simulink model "A"  (Simulink 8.8)
settings: Solver=ode4  StartTime=0.0  StopTime=inf  FixedStep=0.001  RelTol=1e-3  EnableMultiTasking=on
undefined symbols (not defined in the file): mdaadlink6208
settings Model: Creator=Tao  LastModifiedBy=youcaihua  SimulationMode=external
settings SolverCC: EnableConcurrentExecution=on
settings DataIOCC: SaveFormat=StructureWithTime
settings OptimizationCC: BlockReduction=off  OptimizeBlockIOStorage=off  BufferReuse=off  GlobalBufferReuse=off  ExpressionFolding=off  ExpressionDepthLimit=2147483647  LocalBlockOutputs=off  LifeSpan=auto
settings DebuggingCC: SolverPrmCheckMsg=warning
settings HardwareCC: ProdIntDivRoundTo=Zero  ProdEndianess=LittleEndian  ProdLongLongMode=on  ProdHWDeviceType=Generic->32-bit x86 compatible
settings RTWCC: SystemTargetFile=slrt.tlc  TemplateMakefile=slrt_default_tmf  Description=Simulink Real-Time  RTWCompilerOptimization=on

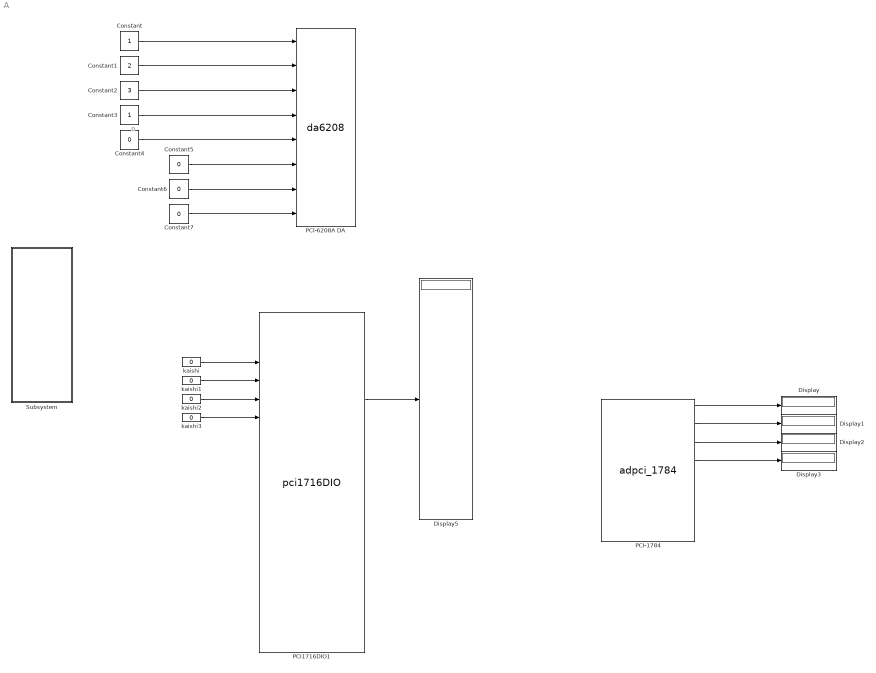
== system A ==
  note: 0
  Constant : Constant
  Constant1 : Constant  Value=2
  Constant2 : Constant  Value=3
  Constant3 : Constant
  Constant{4..7} (4 alike) : Constant  Value=0
  Display{,1..3,5} (5 alike) : Display
  PCI-1784 : S-Function  FunctionName=adpci_1784  Parameters=channel, sampletime, slot  SFunctionDeploymentMode=off  EnableBusSupport=off  mask(PCI-1784){channel=[1 2 3 4 5 6 7 8], sampletime=-1, slot=-1}
      mask prompts: channel "Channel vector:"; sampletime "Sample time:"; slot "PCI slot:"
      mask help:
      | YANHUA
      | PCI-1784
      | Motor Counter
      | UESTC
      mask init:
      | [maskdisplay] = mCntPCI_1784(channel, slot);
      | set_param( gcb, 'MaskDisplay', maskdisplay );
      settings: CopyFcn=|
      | if ~strcmp(get_param(gcb,'Linkstatus'),'none') && ...
      | ~strcmp(get_param(gcb,'Linkstatus'),'implicit')
      |   set_param(gcb,'LinkStatus','none');
      | end
      mask Display: disp('PCI-1784\nUESTC\nMotor Counter');port_label('output',1,'Cnt1');port_label('output',2,'Cnt2');port_label('output',3,'Cnt3');port_label('output',4,'Cnt4');port_label('output',5,'Index1');port_label('output',6,'Index2');port_label('output',7,'Index3');port_label('output',8,'Index4');
  "PCI-6208A DA " : S-Function  InitFcn=mdaadlink6208( 1 );  FunctionName=da6208  Parameters=channel, range, sampletime, pcislot, reset, initval  SFunctionDeploymentMode=off  EnableBusSupport=off  mask(da6208){channel=[1:8], range=4 to 20 ma, reset=[0], initval=[0], sampletime=-1, pcislot=-1}
      mask prompts: channel "Channel vector:"; reset "Reset vector:"; initval "Initial value vector:"; sampletime "Sample time:"; pcislot "PCI slot (-1: autosearch):"
      mask help:
      | PCI-6208A
      | Adlink
      | Analog Output
      mask init:
      | [maskdisplay, reset, initval]= mdaadlink6208(2, channel, reset, initval, pcislot);
      | set_param(gcb,'MaskDisplay',maskdisplay);
      mask Help: helpview(fullfile(docroot, 'mapfiles', 'xpc.map'), 'Adlink_6208A_DA')
      mask TypeOptions range: 0 to 20 ma | 5 to 25 ma | 4 to 20 ma
      mask Display: disp('PCI-6208A\nAdlink\nAnalog Output');port_label('input',1,'1');port_label('input',2,'2');port_label('input',3,'3');port_label('input',4,'4');port_label('input',5,'5');port_label('input',6,'6');port_label('input',7,'7');port_label('input',8,'8');
  PCI1716DIO1 : S-Function  FunctionName=pci1716DIO  Parameters=[SampleTime SampleOffset], SLOT  SFunctionDeploymentMode=off  EnableBusSupport=off  mask{Sample=-1, SLOT=[2 12]}
      mask prompts: Sample "Sample Time:"
      mask help:
      | PCI1716DIO
      | A/D Card
      | Harbin
      | 2014.06.06
      mask init:
      | SampleTime = -1; SampleOffset=0;
      mask Display:
      | disp('PCI1716   A/D&D/A&DIO  ');
      | port_label('input',1 , 'IN1');
      | port_label('input',2 , 'IN2');
      | port_label('input',3 , 'D1');
      | port_label('input',4 , 'D2');
      | port_label('input',5 , 'D3');
      | port_label('input',6 , 'D4');
      | port_label('input',7 , 'D5');
      | port_label('input',8 , 'D6');
      | port_label('input',9 , 'D7');
      | port_label('input',10 , 'D8');
      | port_label('input',11 , 'D9');
      | port_label('input',12 , 'D10');
      | port_label('input',13 , 'D11');
      | port_label('input',14 , 'D12');
      | port_label('input',15 , 'D13');
      | port_label('input',16 , 'D14');
      | port_label('input',17 , 'D15');
      | port_label('input',18, 'D16');
      | port_label('output',1 , 'AD(16)');
      | port_label('output',2 , 'D_OUT(16)');
  Subsystem : Subsystem
  kaishi{,1..3} (4 alike) : Constant  Value=0
      settings: OpenFcn=|
      | if get_param(gcb,'value')=='1',
      | set_param(gcb,'value','0');
      | else
      | set_param(gcb,'value','1');end
  wires:
  PCI-1784/1 -> Display/1
  PCI-1784/2 -> Display1/1
  PCI-1784/3 -> Display2/1
  PCI-1784/4 -> Display3/1
  kaishi/1 -> PCI1716DIO1/3
  kaishi1/1 -> PCI1716DIO1/4
  kaishi2/1 -> PCI1716DIO1/5
  kaishi3/1 -> PCI1716DIO1/6
  PCI1716DIO1/1 -> Display5/1
  Constant/1 -> "PCI-6208A DA "/1
  Constant4/1 -> "PCI-6208A DA "/5
  Constant5/1 -> "PCI-6208A DA "/6
  Constant6/1 -> "PCI-6208A DA "/7
  Constant7/1 -> "PCI-6208A DA "/8
  Constant1/1 -> "PCI-6208A DA "/2
  Constant2/1 -> "PCI-6208A DA "/3
  Constant3/1 -> "PCI-6208A DA "/4

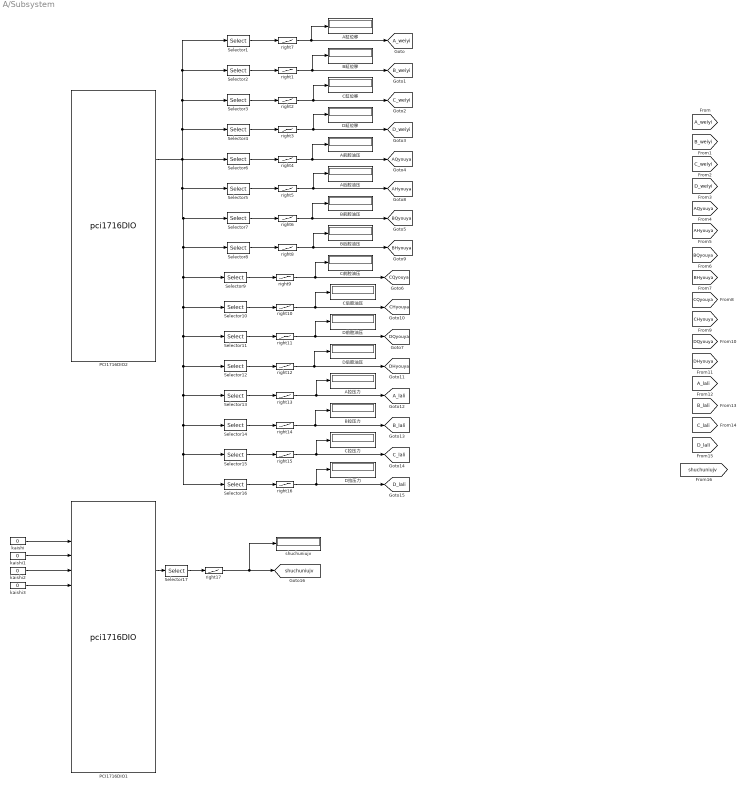
== system A/Subsystem ==
  A前腔油压 : Display
  A后腔油压 : Display
  A拉压力 : Display
  A缸位移 : Display
  B前腔油压 : Display
  B后腔油压 : Display
  B拉压力 : Display
  B缸位移 : Display
  C前腔油压 : Display
  C后腔油压 : Display
  C拉压力 : Display
  C缸位移 : Display
  D前腔油压 : Display
  D后腔油压 : Display
  D拉压力 : Display
  D缸位移 : Display
  PCI1716DIO1 : S-Function  FunctionName=pci1716DIO  Parameters=[SampleTime SampleOffset], SLOT  SFunctionDeploymentMode=off  EnableBusSupport=off  mask{Sample=-1, SLOT=[2 12]}
      mask prompts: Sample "Sample Time:"
      mask help:
      | PCI1716DIO
      | A/D Card
      | Harbin
      | 2014.06.06
      mask init:
      | SampleTime = -1; SampleOffset=0;
      mask Display:
      | disp('PCI1716   A/D&D/A&DIO  ');
      | port_label('input',1 , 'IN1');
      | port_label('input',2 , 'IN2');
      | port_label('input',3 , 'D1');
      | port_label('input',4 , 'D2');
      | port_label('input',5 , 'D3');
      | port_label('input',6 , 'D4');
      | port_label('input',7 , 'D5');
      | port_label('input',8 , 'D6');
      | port_label('input',9 , 'D7');
      | port_label('input',10 , 'D8');
      | port_label('input',11 , 'D9');
      | port_label('input',12 , 'D10');
      | port_label('input',13 , 'D11');
      | port_label('input',14 , 'D12');
      | port_label('input',15 , 'D13');
      | port_label('input',16 , 'D14');
      | port_label('input',17 , 'D15');
      | port_label('input',18, 'D16');
      | port_label('output',1 , 'AD(16)');
      | port_label('output',2 , 'D_OUT(16)');
  PCI1716DIO2 : S-Function  FunctionName=pci1716DIO  Parameters=[SampleTime SampleOffset], SLOT  SFunctionDeploymentMode=off  EnableBusSupport=off  mask{Sample=-1, SLOT=[2 14]}
      mask prompts: Sample "Sample Time:"
      mask help:
      | PCI1716DIO
      | A/D Card
      | Harbin
      | 2014.06.06
      mask init:
      | SampleTime = -1; SampleOffset=0;
      mask Display:
      | disp('PCI1716   A/D&D/A&DIO  ');
      | port_label('input',1 , 'IN1');
      | port_label('input',2 , 'IN2');
      | port_label('input',3 , 'D1');
      | port_label('input',4 , 'D2');
      | port_label('input',5 , 'D3');
      | port_label('input',6 , 'D4');
      | port_label('input',7 , 'D5');
      | port_label('input',8 , 'D6');
      | port_label('input',9 , 'D7');
      | port_label('input',10 , 'D8');
      | port_label('input',11 , 'D9');
      | port_label('input',12 , 'D10');
      | port_label('input',13 , 'D11');
      | port_label('input',14 , 'D12');
      | port_label('input',15 , 'D13');
      | port_label('input',16 , 'D14');
      | port_label('input',17 , 'D15');
      | port_label('input',18, 'D16');
      | port_label('output',1 , 'AD(16)');
      | port_label('output',2 , 'D_OUT(16)');
  Selector1 : Selector  IndexOptions=Index vector (dialog)  Indices=1  OutputSizes=[(-2)]
  Selector10 : Selector  IndexOptions=Index vector (dialog)  Indices=10  OutputSizes=[(-2)]
  Selector11 : Selector  IndexOptions=Index vector (dialog)  Indices=11  OutputSizes=[(-2)]
  Selector12 : Selector  IndexOptions=Index vector (dialog)  Indices=12  OutputSizes=[(-2)]
  Selector13 : Selector  IndexOptions=Index vector (dialog)  Indices=13  OutputSizes=[(-2)]
  Selector14 : Selector  IndexOptions=Index vector (dialog)  Indices=14  OutputSizes=[(-2)]
  Selector15 : Selector  IndexOptions=Index vector (dialog)  Indices=15  OutputSizes=[(-2)]
  Selector16 : Selector  IndexOptions=Index vector (dialog)  Indices=16  OutputSizes=[(-2)]
  Selector17 : Selector  IndexOptions=Index vector (dialog)  Indices=5  OutputSizes=[(-2)]
  Selector2 : Selector  IndexOptions=Index vector (dialog)  Indices=2  OutputSizes=[(-2)]
  Selector3 : Selector  IndexOptions=Index vector (dialog)  Indices=3  OutputSizes=[(-2)]
  Selector4 : Selector  IndexOptions=Index vector (dialog)  Indices=4  OutputSizes=[(-2)]
  Selector5 : Selector  IndexOptions=Index vector (dialog)  Indices=6  OutputSizes=[(-2)]
  Selector6 : Selector  IndexOptions=Index vector (dialog)  Indices=5  OutputSizes=[(-2)]
  Selector7 : Selector  IndexOptions=Index vector (dialog)  Indices=7  OutputSizes=[(-2)]
  Selector8 : Selector  IndexOptions=Index vector (dialog)  Indices=8  OutputSizes=[(-2)]
  Selector9 : Selector  IndexOptions=Index vector (dialog)  Indices=9  OutputSizes=[(-2)]
  kaishi{,1..3} (4 alike) : Constant  Value=0
      settings: OpenFcn=|
      | if get_param(gcb,'value')=='1',
      | set_param(gcb,'value','0');
      | else
      | set_param(gcb,'value','1');end
  right{1..3,7} (4 alike) : Lookup  InputValues=[0 10]  Table=[0 25]  SaturateOnIntegerOverflow=on
  right{4..6,8..12} (8 alike) : Lookup  InputValues=[0 10]  Table=[0 10]  SaturateOnIntegerOverflow=on
  right{13..16} (4 alike) : Lookup  InputValues=[0 10]  Table=[-5000 5000]  SaturateOnIntegerOverflow=on
  right17 : Lookup  InputValues=[0 10]  Table=[-1500 1500]  SaturateOnIntegerOverflow=on
  shuchuniujv : Display
  tag scope: AHyouya=global, AQyouya=global, A_lali=global, A_weiyi=global, BHyouya=global, BQyouya=global, B_lali=global, B_weiyi=global, CHyouya=global, CQyouya=global, C_lali=global, C_weiyi=global, DHyouya=global, DQyouya=global, D_lali=global, D_weiyi=global, shuchuniujv=global
  wires:
  PCI1716DIO2/1 -> Selector6/1, Selector4/1, Selector3/1, Selector2/1, Selector1/1, Selector16/1, Selector15/1, Selector14/1, Selector13/1, Selector12/1, Selector11/1, Selector10/1, Selector9/1, Selector8/1, Selector7/1, Selector5/1
  Selector1/1 -> right7/1
  right7/1 -> A缸位移/1, [A_weiyi]
  Selector4/1 -> right3/1
  Selector3/1 -> right2/1
  Selector2/1 -> right1/1
  right1/1 -> B缸位移/1, [B_weiyi]
  right2/1 -> C缸位移/1, [C_weiyi]
  right3/1 -> D缸位移/1, [D_weiyi]
  Selector6/1 -> right4/1
  Selector5/1 -> right5/1
  Selector7/1 -> right6/1
  Selector8/1 -> right8/1
  Selector9/1 -> right9/1
  Selector10/1 -> right10/1
  Selector11/1 -> right11/1
  Selector12/1 -> right12/1
  Selector13/1 -> right13/1
  Selector14/1 -> right14/1
  Selector15/1 -> right15/1
  Selector16/1 -> right16/1
  right4/1 -> A前腔油压/1, [AQyouya]
  right6/1 -> B前腔油压/1, [BQyouya]
  right9/1 -> C前腔油压/1, [CQyouya]
  right11/1 -> D前腔油压/1, [DQyouya]
  right5/1 -> A后腔油压/1, [AHyouya]
  right8/1 -> B后腔油压/1, [BHyouya]
  right10/1 -> C后腔油压/1, [CHyouya]
  right12/1 -> D后腔油压/1, [DHyouya]
  right13/1 -> A拉压力/1, [A_lali]
  right14/1 -> B拉压力/1, [B_lali]
  right15/1 -> C拉压力/1, [C_lali]
  right16/1 -> D拉压力/1, [D_lali]
  kaishi/1 -> PCI1716DIO1/3
  kaishi1/1 -> PCI1716DIO1/4
  kaishi2/1 -> PCI1716DIO1/5
  kaishi3/1 -> PCI1716DIO1/6
  PCI1716DIO1/1 -> Selector17/1
  Selector17/1 -> right17/1
  right17/1 -> shuchuniujv/1, [shuchuniujv]
